simulink model "xiti4_8_10T1"  (Simulink 5.0)
settings: Solver=ode45  StartTime=0.0  StopTime=20  FixedStep=0.01  RelTol=1e-3
libraries: simulink_extras x2
CloseFcn:
  | rtwprivate ssgensfun ModelCloseRequest PID_PI
settings Model: LastModifiedBy=ThinkPad

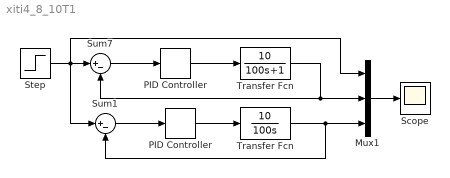
== system xiti4_8_10T1 ==
  Mux1 : Mux  Inputs=3
  PID Controller : simulink_extras/Additional Linear/PID Controller  P=10  I=0  D=0
  "PID Controller " : simulink_extras/Additional Linear/PID Controller  P=10  I=0  D=0
  "Scope " : Scope
      settings: YMin=0  YMax=1.5  SaveName=xiti4_81  DataFormat=Array  MaxDataPoints=500000
  Step : Step  Time=0  SampleTime=0
  Sum1 : Sum  Inputs=|+-  SaturateOnIntegerOverflow=on
  Sum7 : Sum  Inputs=|+-  SaturateOnIntegerOverflow=on
  Transfer Fcn : TransferFcn  Numerator=[10]  Denominator=[100 1]
  "Transfer Fcn " : TransferFcn  Numerator=[10]  Denominator=[100 0]
  wires:
  Step/1 -> Sum7/1, Sum1/1, Mux1/1
  Sum7/1 -> "PID Controller "/1
  "PID Controller "/1 -> Transfer Fcn/1
  Transfer Fcn/1 -> Sum7/2, Mux1/2
  Sum1/1 -> PID Controller/1
  PID Controller/1 -> "Transfer Fcn "/1
  "Transfer Fcn "/1 -> Sum1/2, Mux1/3
  Mux1/1 -> "Scope "/1
